simulink model "tasks_union_1"  (R2020b)
settings: Solver=FixedStepAuto  StartTime=0.0  StopTime=5  FixedStep=0.001  RelTol=1e-3
values from neighbouring files (symbols this model uses):
  a = evalin('base','a')    [Coriolis.m]    (also in init.m = 0.5)
  a0 = 0.99    [init.m]
  ac = mass_can*(l1*l2)    (= 0.5)    [init.m]
  berta = 0.98    [init.m]
  csi = 1    [init.m]
  e_max = 0.01    [init.m]
  F_int_max = [2;2]    [init.m]
  F_max = [2;2]    [init.m]
  F_weight = [0;-0.5*mass_can*g]    [init.m]
  g = evalin('base','g')    [Gravity.m]    (also in init.m = 9.81)
  I1 = evalin('base','I1')    [Mass.m]    (also in init.m = 1)
  I2 = evalin('base','I2')    [Mass.m]    (also in init.m = 1)
  Ic = mass_can*l2^2    (= 0.5)    [init.m]
  l1 = evalin('base','l1')    [Gravity.m]    (also in Jacobianoa_dot.m; Mass.m; cin_dir.m; init.m = 1)
  l2 = evalin('base','l2')    [Gravity.m]    (also in Jacobianoa_dot.m; Mass.m; cin_dir.m; init.m = 1)
  M = 0.1    [init.m]
  m1 = evalin('base','m1')    [Gravity.m]    (also in Mass.m; init.m = 1)
  m2 = evalin('base','m2')    [Gravity.m]    (also in Mass.m; init.m = 1)
  mass = 0.1    [init.m]
  mass_can = 0.5    [init.m]
libraries: simulink x1
settings Model: Creator=chiara-s  LastModifiedBy=chiara-s

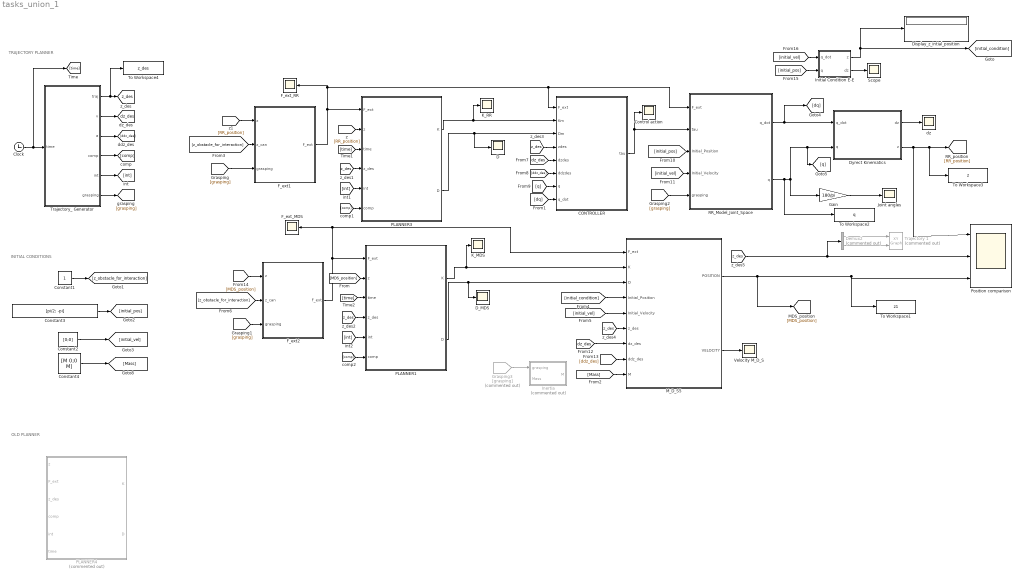
== system tasks_union_1 ==
  note: OLD PLANNER
  note: TRAJECTORY PLANNER
  note: INITIAL CONDITIONS
  CONTROLLER : MATLAB Function  TreatAsAtomicUnit=on
  Clock : Clock
  Constant1 : Constant
  Constant2 : Constant  Value=[0;0]
  Constant3 : Constant  Value=[pi/2; -pi]
  Constant4 : Constant  Value=[M 0;0 M]
  Control action : Scope
  D : Scope
  D_MDS : Scope
  Demux2 : Demux  Commented=on  Outputs=2
  Display_z_intial_position : Display
  Dyrect Kinematics : MATLAB Function  TreatAsAtomicUnit=on
  F_ext1 : MATLAB Function  TreatAsAtomicUnit=on
  F_ext2 : MATLAB Function  TreatAsAtomicUnit=on
  F_ext_MDS : Scope
  F_ext_RR : Scope
  Gain : Gain  Gain=180/pi
  Grasping3 : From  Commented=on  GotoTag=grasping
  "Inertia " : MATLAB Function  Commented=on  TreatAsAtomicUnit=on
  Initial Condition E-E : MATLAB Function  TreatAsAtomicUnit=on
  Joint angles : Scope
  K_MDS : Scope
  K_RR : Scope
  M_D_S5 : Subsystem
  PLANNER1 : Subsystem
  PLANNER3 : Subsystem
  PLANNER4 : Subsystem  Commented=on
  Position comparison : Scope  NumInputPorts=3
  RR_Model_Joint_Space : Subsystem
  Scope : Scope
  To Workspace1 : ToWorkspace  VariableName=z1  SaveFormat=Timeseries  SampleTime=-1
  To Workspace2 : ToWorkspace  VariableName=q  SaveFormat=Timeseries  SampleTime=-1
      settings: Save2DSignal=2-D array (concatenate along first dimension)
  To Workspace3 : ToWorkspace  VariableName=z  SaveFormat=Timeseries  SampleTime=-1
  To Workspace4 : ToWorkspace  VariableName=z_des  SaveFormat=Timeseries  SampleTime=-1
      settings: Save2DSignal=2-D array (concatenate along first dimension)
  Trajectory 1 : simulink/Sinks/XY Graph  Commented=on  xmin=-2  xmax=2  ymin=-2  ymax=2  st=-1
  Trajectory_ Generator : MATLAB Function  TreatAsAtomicUnit=on
  Velocity M_D_S : Scope
  dz : Scope
  tag scope: dz_des=global, z_des=global
  wires:
  Initial Condition E-E/1(z) -> Display_z_intial_position/1, [initial_condition]
  Initial Condition E-E/2(dz) -> Scope/1
  Gain/1 -> Joint angles/1
  Constant1/1 -> [z_obstacle_for_interaction]
  Constant2/1 -> [initial_vel]
  Constant3/1 -> [initial_pos]
  Constant4/1 -> [Mass]
  Clock/1 -> [time], Trajectory_ Generator/1(time)
  [z_obstacle_for_interaction] -> F_ext2/2(z_can)
  Trajectory_ Generator/1(traj) -> To Workspace4/1, [z_des]
  Trajectory_ Generator/2(v) -> [dz_des]
  Trajectory_ Generator/3(a) -> [ddz_des]
  Trajectory_ Generator/4(comp) -> [comp]
  Trajectory_ Generator/5(int) -> [int]
  Trajectory_ Generator/6(grasping) -> [grasping]
  [grasping] -> F_ext1/3(grasping)
  [grasping] -> F_ext2/3(grasping)
  [time] -> PLANNER3/3(time)
  [z_des] -> PLANNER1/4(z_des)
  [z_obstacle_for_interaction] -> F_ext1/2(z_can)
  [comp] -> PLANNER1/6(comp)
  [int] -> PLANNER3/5(int)
  [int] -> PLANNER1/5(int)
  [time] -> PLANNER1/3(time)
  RR_Model_Joint_Space/1(q_dot) -> [dq], Dyrect Kinematics/1(q_dot)
  RR_Model_Joint_Space/2(q) -> Gain/1, [q], Dyrect Kinematics/2(q), To Workspace2/1
  Dyrect Kinematics/1(dz) -> dz/1
  Dyrect Kinematics/2(z) -> Position comparison/1, To Workspace3/1, [RR_position]
  F_ext1/1(F_ext) -> PLANNER3/1(F_ext), RR_Model_Joint_Space/1(F_ext), CONTROLLER/1(F_ext), F_ext_RR/1
  [RR_position] -> F_ext1/1(z)
  CONTROLLER/1(tau) -> Control action/1, RR_Model_Joint_Space/2(tau)
  [z_des] -> CONTROLLER/4(zdes)
  [dz_des] -> CONTROLLER/5(dzdes)
  PLANNER3/1(K) -> K_RR/1, CONTROLLER/2(Km)
  PLANNER3/2(D) -> D/1, CONTROLLER/3(Dm)
  PLANNER1/1(K) -> K_MDS/1, M_D_S5/2(K)
  PLANNER1/2(D) -> D_MDS/1, M_D_S5/3(D)
  [ddz_des] -> CONTROLLER/6(ddzdes)
  [initial_pos] -> RR_Model_Joint_Space/3(Initial_Position)
  [initial_vel] -> RR_Model_Joint_Space/4(Initial_Velocity)
  [grasping] -> RR_Model_Joint_Space/5(grasping)
  [initial_condition] -> M_D_S5/4(Initial_Position)
  [initial_vel] -> M_D_S5/5(Initial_Velocity)
  Grasping3/1 -> "Inertia "/1(grasping)
  [z_des] -> M_D_S5/6(z_des)
  [dz_des] -> M_D_S5/7(dz_des)
  [ddz_des] -> M_D_S5/8(ddz_des)
  M_D_S5/2(VELOCITY) -> Velocity M_D_S/1
  M_D_S5/1(POSITION) -> [MDS_position], To Workspace1/1, Position comparison/3
  [z_des] -> Demux2/1, Position comparison/2
  Demux2/2 -> Trajectory 1/2
  Demux2/1 -> Trajectory 1/1
  [dq] -> CONTROLLER/8(q_dot)
  [q] -> CONTROLLER/7(q)
  [MDS_position] -> F_ext2/1(z)
  [initial_vel] -> Initial Condition E-E/1(q_dot)
  [initial_pos] -> Initial Condition E-E/2(q)
  F_ext2/1(F_ext) -> PLANNER1/1(F_ext), M_D_S5/1(F_ext), F_ext_MDS/1
  [Mass] -> M_D_S5/9(M)
  [RR_position] -> PLANNER3/2(z)
  [comp] -> PLANNER3/6(comp)
  [z_des] -> PLANNER3/4(z_des)
  [MDS_position] -> PLANNER1/2(z)

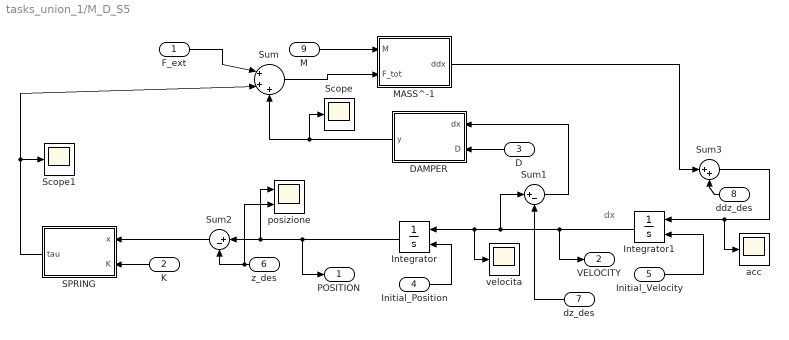
== system tasks_union_1/M_D_S5 ==
  note: dx
  F_ext : Inport
  K : Inport  Port=2
  D : Inport  Port=3
  Initial_Position : Inport  Port=4
  Initial_Velocity : Inport  Port=5
  z_des : Inport  Port=6
  dz_des : Inport  Port=7
  ddz_des : Inport  Port=8
  M : Inport  Port=9
  DAMPER : MATLAB Function  TreatAsAtomicUnit=on
  Integrator : Integrator  InitialConditionSource=external
  Integrator1 : Integrator  InitialConditionSource=external
  MASS^-1 : MATLAB Function  TreatAsAtomicUnit=on
  SPRING : MATLAB Function  TreatAsAtomicUnit=on
  Scope : Scope
  Scope1 : Scope
  Sum : Sum  Inputs=|+++
  Sum1 : Sum  Inputs=|+-
  Sum2 : Sum  Inputs=|+-
  Sum3 : Sum  Inputs=|++
  acc : Scope
  posizione : Scope  NumInputPorts=2
  velocita : Scope
  POSITION : Outport
  VELOCITY : Outport  Port=2
  wires:
  Integrator1/1 -> velocita/1, Integrator/1, Sum1/1, VELOCITY/1
  SPRING/1(tau) -> Sum/2, Scope1/1
  Integrator/1 -> posizione/1, Sum2/1, POSITION/1
  DAMPER/1(y) -> Scope/1, Sum/3
  Sum/1 -> MASS^-1/2(F_tot)
  M/1 -> MASS^-1/1(M)
  D/1 -> DAMPER/2(D)
  K/1 -> SPRING/2(K)
  Initial_Velocity/1 -> Integrator1/2
  Initial_Position/1 -> Integrator/2
  z_des/1 -> posizione/2, Sum2/2
  Sum2/1 -> SPRING/1(x)
  MASS^-1/1(ddx) -> Sum3/1
  Sum1/1 -> DAMPER/1(dx)
  Sum3/1 -> acc/1, Integrator1/1
  dz_des/1 -> Sum1/2
  ddz_des/1 -> Sum3/2
  F_ext/1 -> Sum/1

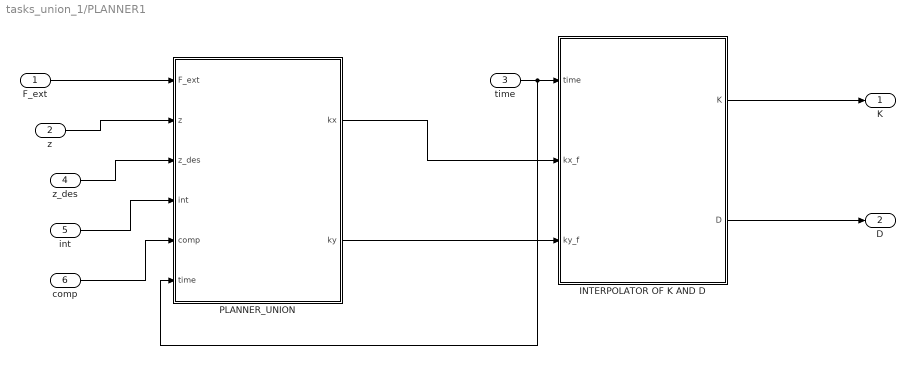
== system tasks_union_1/PLANNER1 ==
  F_ext : Inport
  z : Inport  Port=2
  time : Inport  Port=3
  z_des : Inport  Port=4
  int : Inport  Port=5
  comp : Inport  Port=6
  "INTERPOLATOR OF K AND D " : MATLAB Function  TreatAsAtomicUnit=on
  PLANNER_UNION : MATLAB Function  TreatAsAtomicUnit=on
  K : Outport
  D : Outport  Port=2
  wires:
  time/1 -> "INTERPOLATOR OF K AND D "/1(time), PLANNER_UNION/6(time)
  "INTERPOLATOR OF K AND D "/2(D) -> D/1
  "INTERPOLATOR OF K AND D "/1(K) -> K/1
  PLANNER_UNION/2(ky) -> "INTERPOLATOR OF K AND D "/3(ky_f)
  PLANNER_UNION/1(kx) -> "INTERPOLATOR OF K AND D "/2(kx_f)
  int/1 -> PLANNER_UNION/4(int)
  comp/1 -> PLANNER_UNION/5(comp)
  F_ext/1 -> PLANNER_UNION/1(F_ext)
  z/1 -> PLANNER_UNION/2(z)
  z_des/1 -> PLANNER_UNION/3(z_des)

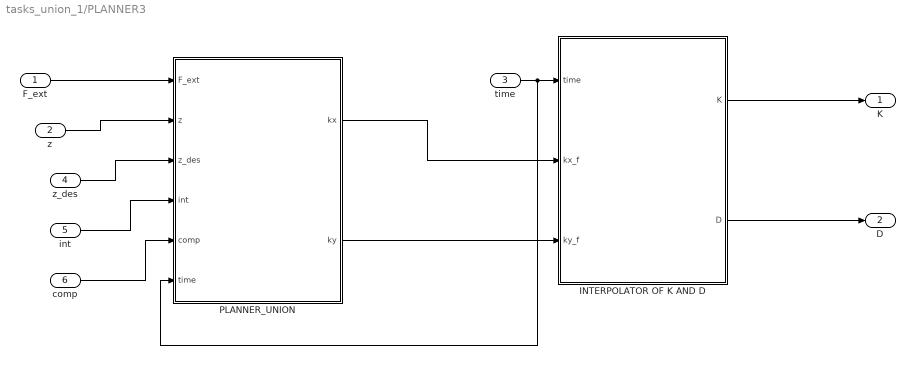
== system tasks_union_1/PLANNER3 ==
  F_ext : Inport
  z : Inport  Port=2
  time : Inport  Port=3
  z_des : Inport  Port=4
  int : Inport  Port=5
  comp : Inport  Port=6
  "INTERPOLATOR OF K AND D " : MATLAB Function  TreatAsAtomicUnit=on
  PLANNER_UNION : MATLAB Function  TreatAsAtomicUnit=on
  K : Outport
  D : Outport  Port=2
  wires:
  time/1 -> "INTERPOLATOR OF K AND D "/1(time), PLANNER_UNION/6(time)
  "INTERPOLATOR OF K AND D "/2(D) -> D/1
  "INTERPOLATOR OF K AND D "/1(K) -> K/1
  PLANNER_UNION/2(ky) -> "INTERPOLATOR OF K AND D "/3(ky_f)
  PLANNER_UNION/1(kx) -> "INTERPOLATOR OF K AND D "/2(kx_f)
  int/1 -> PLANNER_UNION/4(int)
  comp/1 -> PLANNER_UNION/5(comp)
  F_ext/1 -> PLANNER_UNION/1(F_ext)
  z/1 -> PLANNER_UNION/2(z)
  z_des/1 -> PLANNER_UNION/3(z_des)

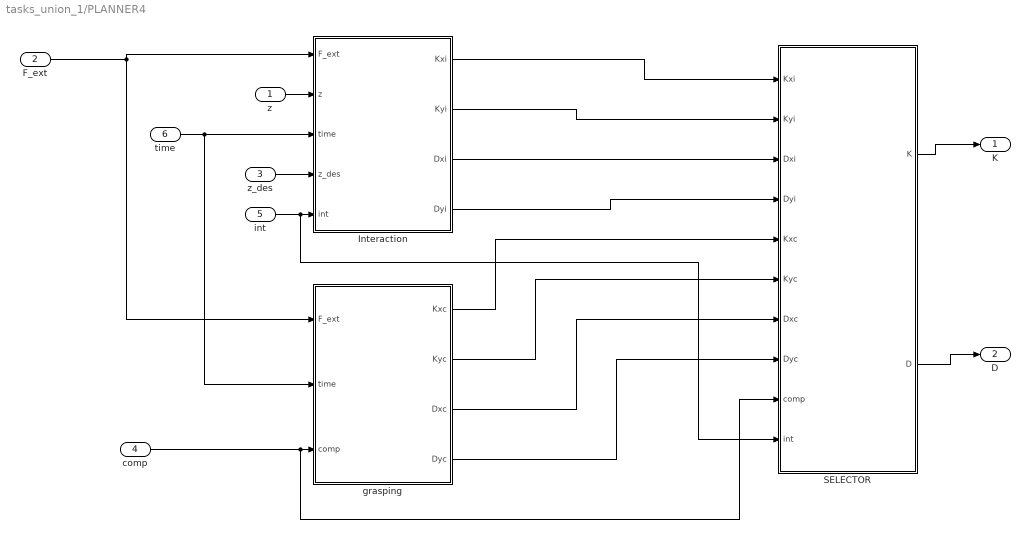
== system tasks_union_1/PLANNER4 ==
  z : Inport
  F_ext : Inport  Port=2
  z_des : Inport  Port=3
  comp : Inport  Port=4
  int : Inport  Port=5
  time : Inport  Port=6
  Interaction : MATLAB Function  TreatAsAtomicUnit=on
  SELECTOR : MATLAB Function  TreatAsAtomicUnit=on
  grasping : MATLAB Function  TreatAsAtomicUnit=on
  K : Outport
  D : Outport  Port=2
  wires:
  time/1 -> grasping/2(time), Interaction/3(time)
  z_des/1 -> Interaction/4(z_des)
  F_ext/1 -> grasping/1(F_ext), Interaction/1(F_ext)
  z/1 -> Interaction/2(z)
  SELECTOR/1(K) -> K/1
  SELECTOR/2(D) -> D/1
  Interaction/1(Kxi) -> SELECTOR/1(Kxi)
  Interaction/2(Kyi) -> SELECTOR/2(Kyi)
  Interaction/3(Dxi) -> SELECTOR/3(Dxi)
  Interaction/4(Dyi) -> SELECTOR/4(Dyi)
  grasping/1(Kxc) -> SELECTOR/5(Kxc)
  grasping/2(Kyc) -> SELECTOR/6(Kyc)
  grasping/3(Dxc) -> SELECTOR/7(Dxc)
  grasping/4(Dyc) -> SELECTOR/8(Dyc)
  comp/1 -> SELECTOR/9(comp), grasping/3(comp)
  int/1 -> SELECTOR/10(int), Interaction/5(int)

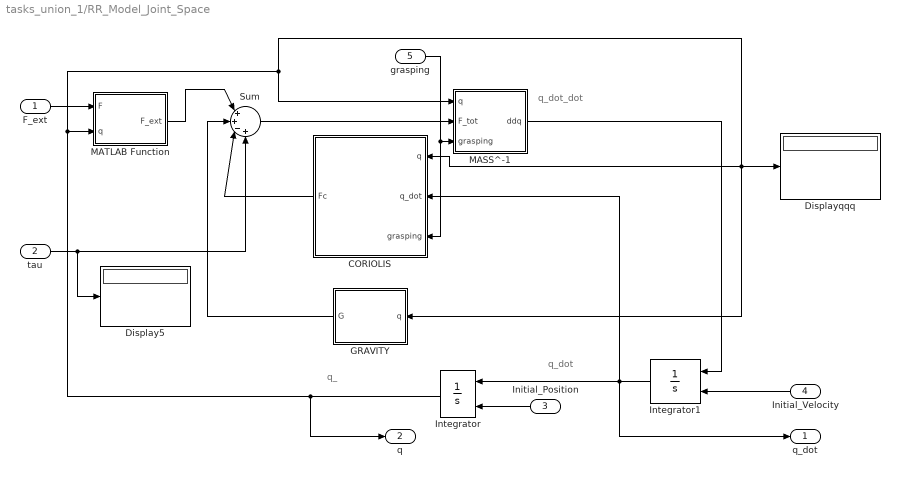
== system tasks_union_1/RR_Model_Joint_Space ==
  note: q_dot
  note: q_dot_dot
  note: q_
  F_ext : Inport
  tau : Inport  Port=2
  Initial_Position : Inport  Port=3
  Initial_Velocity : Inport  Port=4
  grasping : Inport  Port=5
  CORIOLIS : MATLAB Function  TreatAsAtomicUnit=on
  Display5 : Display
  Displayqqq : Display
  GRAVITY : MATLAB Function  TreatAsAtomicUnit=on
  Integrator : Integrator  InitialConditionSource=external
  Integrator1 : Integrator  InitialConditionSource=external  InitialCondition=[0;0]
  MASS^-1 : MATLAB Function  TreatAsAtomicUnit=on
  MATLAB Function : MATLAB Function  TreatAsAtomicUnit=on
  Sum : Sum  Inputs=|++-+
  q_dot : Outport
  q : Outport  Port=2
  wires:
  GRAVITY/1(G) -> Sum/2
  MATLAB Function/1(F_ext) -> Sum/1
  Initial_Position/1 -> Integrator/2
  F_ext/1 -> MATLAB Function/1(F)
  Integrator/1 -> MASS^-1/1(q), GRAVITY/1(q), Displayqqq/1, CORIOLIS/1(q), MATLAB Function/2(q), q/1
  Integrator1/1 -> q_dot/1, CORIOLIS/2(q_dot), Integrator/1
  Initial_Velocity/1 -> Integrator1/2
  MASS^-1/1(ddq) -> Integrator1/1
  Sum/1 -> MASS^-1/2(F_tot)
  CORIOLIS/1(Fc) -> Sum/3
  tau/1 -> Display5/1, Sum/4
  grasping/1 -> CORIOLIS/3(grasping), MASS^-1/3(grasping)

== matlab function tasks_union_1/Dyrect Kinematics ==
  data: q_dot input double size=2; dz output double size=2; q input double size=2; z output double size=2; l1 parameter; l2 parameter
function [dz,z] = fcn(q_dot,q,l1, l2)

z = zeros(2,1);
z(1) = l1*cos(q(1)) + l2*cos(q(1)+q(2));
z(2) = l1*sin(q(1)) + l2*sin(q(1)+q(2));

Ja = zeros(2,2);
Ja = [-l1*sin(q(1)) - l2*sin(q(1)+q(2)), -l2*sin(q(1)+q(2)); ...
    l1*cos(q(1)) + l2*cos(q(1)+q(2)), l2*cos(q(1)+q(2))];

dz = zeros(2,1);
dz = Ja*q_dot;

end

== matlab function tasks_union_1/PLANNER1/PLANNER_UNION ==
  settings: updateMethod=DISCRETE
  data: kx output; F_ext input; z input; z_des input; int input; comp input; ky output; e_max parameter; F_max parameter; F_int_max parameter; time input
function [kx, ky] = fcn(F_ext, z, z_des, int, comp, e_max, F_max, F_int_max, time)
%% Description MDS_interaction


%% Outputs
% K            stiffness 
% D            damping 

%% Inputs
% time          current simulation time
% F_ext         measured external force
% mass          mass scalar value 
% F_int_max     desired interaction force
% z_des         desired trajectory
% z             current position
% F_max         estimated force disturbances
% e_max         maximum steady-state error

persistent kxi kyi kxc kyc F_comp
persistent int_prec comp_prec z_int z_int_dir 

% persistent initialization
if isempty(kxi)
   kxi = F_max(1)/e_max; 
end
if isempty(F_comp)
   F_comp = [0;0];
end

if isempty(kyi)
   kyi = F_max(2)/e_max;
end
if isempty(kxc)
      kxc = F_max(1)/e_max;
end
if isempty(kyc)
      kyc = F_max(2)/e_max;
end
if isempty(z_int) 
    z_int = [1000; 1000];
end
if isempty(z_int_dir) 
    z_int_dir = [0;0];
end
if isempty(int_prec)
    int_prec = [0;0];
end
if isempty(comp_prec)
    comp_prec = [0;0];
end

% interaction X axes
if int(1) == 1
    if abs(F_ext(1)-F_comp(1)) > F_max(1)         % F_max soglia dei disturbi
        if z_int(1) == 1000
            z_int(1) = z(1);
            z_int_dir(1) = -sign(F_ext(1)-F_comp(1));     % direzione non permessa
        end
    end
    if abs(F_ext(1)-F_comp(1)) > F_int_max(1) 
            % if interaction force is higher than threshold
            if kxi*abs(z(1)-z_des(1)) > F_int_max(1)
                % set k 
                ktemp_x = F_int_max(1)/abs(z(1)-z_des(1));
                if ktemp_x < kxi
                    kxi = ktemp_x;
                end
            end
    end
end

% interaction Y axes
if int(2) == 1
    if abs(F_ext(2)-F_comp(2)) > F_max(2)         % F_max soglia dei disturbi
        if z_int(2) == 1000
            z_int(2) = z(2);
            z_int_dir(2) = -sign(F_ext(2)-F_comp(2));     % direzione non permessa
        end
    end
    % Similarly for the other direction
    if abs(F_ext(2)-F_comp(2)) > F_int_max(2) 
            if kyi*abs(z(2)-z_des(2)) > F_int_max(2)
                ktemp_y = F_int_max(2)/abs(z(2)-z_des(2));
                if ktemp_y < kyi
                    kyi = ktemp_y;
                end
            end
    end
end

% compensation X axes
if comp(1) == 1
    if z_int(1) == 1000
       if abs(F_ext(1))/kxc > e_max
            kxc = abs(F_ext(1))/e_max;
            F_comp(1) = F_ext(1);
       end
    else 
        if z_int_dir(1) == 1
            if z(1) < z_int(1)
                if abs(F_ext(1))/kxc > e_max 
                    kxc = abs(F_ext(1))/e_max;
                    F_comp(1) = F_ext(1);
                end
            end
        else
            if z(1) > z_int(1)
                if abs(F_ext(1))/kxc > e_max
                    kxc = abs(F_ext(1))/e_max;
                    F_comp(1) = F_ext(1);
                end
            end
        end
                
   end
end

% compensation Y axes
if comp(2) == 1
    if z_int(2) == 1000 
       if abs(F_ext(2))/kyc > e_max
            kyc = abs(F_ext(2))/e_max;
            F_comp(2) = F_ext(2);
       end
    else 
        if z_int_dir(2) == 1
            if z(2) < z_int(2)
                if abs(F_ext(2))/kyc > e_max
                    kyc = abs(F_ext(2))/e_max;
                    F_comp(2) = F_ext(2);
                end
            end
        else
            if z(2) > z_int(2)
                if abs(F_ext(2))/kyc > e_max
                    kyc = abs(F_ext(2))/e_max;
                    F_comp(2) = F_ext(2);
                end
            end
        end
                
   end
end

% reset to default
if comp(1)==0 && comp_prec(1)==1
%     z_int_dir(1) = 0;
%     z_int(1) = 1000;
    kxc = F_max(1)/e_max;
    F_comp(1) = 0;
end
if comp(2)==0 && comp_prec(2)==1
%     z_int_dir(2) = 0;
%     z_int(2) = 1000;
    kyc = F_max(2)/e_max;
    F_comp(2) = 0;
end
if int(1)==0 && int_prec(1)==1
    kxi = F_max(1)/e_max;
end
if int(2)==0 && int_prec(2)==1
    kyi = F_max(2)/e_max;
end
% quando c'è una interazione e prima non c'era risetto tutto (RACCAPEZZO)
if int(1)==1 && int_prec(1)==0
    if comp_prec(1) == 1
        kxi = kxc;
    end
    z_int(1)=1000;
    z_int_dir(1)=0;
end
if int(2)==1 && int_prec(2)==0
    if comp_prec(2) == 1
        kyi = kyc;
    end
    z_int(2)=1000;
    z_int_dir(2)=0;
end
if comp(1) == 1 && comp_prec(1)==0
    if int_prec(1) == 1
        kxc = kxi;
    end
end
if comp(2) == 1 && comp_prec(2)==0
    if int_prec(2)==1
        kyc =kyi;
    end
end
% update last booleans
int_prec = int;
comp_prec = comp;


% Final Values of D-K
kx = abs(F_max(1))/e_max;
ky = abs(F_max(2))/e_max;

if comp(1) == 1
    kx = kxc;
end
if comp(2) == 1
    ky = kyc;
end
if int(1) == 1
    kx = kxi;
    if comp(1) == 1
        if z_int(1) == 1000
            kx = kxc;
        else
            if z_int_dir(1) == 1
                if z_des(1) < z_int(1)
                    kx = kxc;
                end
            else
                if z_des(1) > z_int(1)
                    kx = kxc;
                end
            end
        end
    else
        if z_int(1) == 1000
            kx = F_max(1)/e_max;
        else
            if z_int_dir(1) == 1
                if z_des(1) < z_int(1)
                    kx = F_max(1)/e_max;
                end
            else
                if z_des(1) > z_int(1)
                    kx = F_max(1)/e_max;
                end
            end
        end
    end
end
if int(2) == 1
    ky = kyi;
     if comp(2) == 1
        if z_int(2) == 1000
            kx = kxc;
        else
            if z_int_dir(2) == 1
                if z_des(2) < z_int(2) 
                    ky = kyc;
                end
            else
                if z_des(2) > z_int(2)
                    ky = kyc;
                end
            end
        end
     else
         if z_int(2) == 1000
            kx = F_max(2)/e_max;
        else
            if z_int_dir(2) == 1
                if z_des(2) < z_int(2) 
                    ky = F_max(2)/e_max;
                end
            else
                if z_des(2) > z_int(2)
                    ky = F_max(2)/e_max;
                end
            end
        end
     end
end

end

== matlab function tasks_union_1/Trajectory_ Generator ==
  data: time input; traj output; v output; a output; comp output; int output; grasping output
function [traj,v, a, comp, int, grasping] = fcn(time)

comp = [0;0];
int = [0;0];
t_prec = 0;
grasping = 0;

if time < 0.1
    a = [5;0];
    traj = 0.5*a*(time)^2;   % initial vel = 0;
    v = a*time;
    int(1) = 1;
elseif time < 2.3
    v = [0.5;0];
    x0 = [0.025;0];
    traj = x0 + v*(time-0.1); 
    a = [0;0];
    int(1) = 1;
elseif time < 2.4
    a = [-5;0];
    x0 = [1.125;0];
    v0 = [0.5;0];
    v = v0 + a*(time -2.3);
    traj = x0 + 0.5*a*(time -2.3)^2 + v0*(time-2.3);
    int(1) = 1;
elseif time < 3
    int(1) = 1;
    traj = [1.15;0];  
    a = [0;0];
    v = [0;0];
elseif time < 3.1
    a = [0; 5];
    v = a*(time-3);
    x0 = [1.15;0];
    traj = 0.5*a*(time -3)^2 + x0;
    comp(2) = 1;
    int(1) = 1;
    grasping = 1;
elseif time < 4.1
    comp(2) = 1;
    v = [0; 0.5];
    x0 = [1.15;0.025];
    traj = x0 + v*(time-3.1);
    a = [0;0];
    grasping = 1;
    int(1) = 1;
elseif time < 4.2
    comp(2) = 1;
    a = [0; -5];
    x0 = [1.15; 0.525];
    v0 = [0; 0.5];
    v = v0 +a*(time-4.1);
    traj = x0 + 0.5*a*(time-4.1)^2 + v0*(time-4.1);
    grasping = 1;
else
    traj = [1.15; 0.55];
    comp(2) = 1;
    a = [0;0];
    v = [0;0];
    grasping = 1;
end

end

== matlab function tasks_union_1/F_ext1 ==
  data: z input; F_ext output; z_can input; grasping input; mass_can parameter; g parameter
function F_ext = fcn(z, z_can, grasping, mass_can, g)
% hypothesis: table reaction force with elastic behaviour
F_ext = zeros(2,1);
k_can = 500;         
k_table = 10000;
% if contact is happened with can
if grasping == 0
    if z(1) > z_can
        F_ext(1) = k_can*(z_can - z(1));    % force to the left
    end
else 
    F_ext(1) = 0;
    F_ext(2) = -mass_can*g;
    if z(2) < 0
         F_ext(2) = - k_table*z(2);       % in grasping on the table
    else 
        if (abs(k_table*z(2)) < abs(mass_can*g))
            F_ext(2) = - k_table*z(2);
        else 
            F_ext(2) = - mass_can*g;        % STACCATO
        end    
    end
end
end

== matlab function tasks_union_1/Inertia  ==
  data: M output; grasping input; mass_can parameter; Mass input
function M = fcn(grasping, mass_can, Mass)

if grasping == 1
    M = diag([Mass(1,1)+mass_can Mass(2,2)+mass_can]);
else
    M = Mass;
end

end

== matlab function tasks_union_1/CONTROLLER ==
  data: F_ext input; Km input; Dm input; zdes input size=2; tau output double size=2; dzdes input size=2; ddzdes input size=2; q input size=2; q_dot input size=2; M parameter
function tau = fcn(F_ext,Km, Dm,zdes, dzdes, ddzdes, q, q_dot, M)
%% PROBLEMA MATRICE DELLE MASSE NON DIAGONALE
coder.extrinsic('Jacobianoa','Jacobianoa_dot','Mass','Coriolis','Gravity','cin_dir')
dz = zeros(2,1);
z = zeros(2,1);
B = zeros(2,2);
S = zeros(2,2);
G = zeros(2,1);
Ja = zeros(2,2);
Ja_dot = zeros(2,2);
Bm = [M 0; 0 M];
Ja = Jacobianoa(q);
Ja_dot = Jacobianoa_dot(q,q_dot);

dz = Ja*q_dot;
z = cin_dir(q);

t = 0.1;
if (deg2rad(-0.1) < q(2)) && (q(2) < deg2rad(0.1)) || (deg2rad(179.9) < q(2)) && (q(2) < deg2rad(180.1)) || (deg2rad(-180.1) < q(2)) && (q(2) < deg2rad(-179.9))
    Ja_inv = (Ja')*inv(Ja*(Ja') + t^2*eye(2,2)); % Damp least square Jacobian method
else 
    Ja_inv = inv(Ja);
end

% Ja_inv = inv(Ja);

B = Mass(q);
Bx = (Ja_inv')* B * Ja_inv;
S = Coriolis(q,q_dot);
G = Gravity(q);
I = eye(2,2);
% tau = B * Ja_inv*(ddzdes - Ja_dot*q_dot) + ...
%     S*q_dot + (Ja')*(Dm*(dzdes - dz) + Km*(zdes- z)) + G;

tau = B*Ja_inv*(ddzdes - Ja_dot*q_dot + ...
    inv(Bm)*(Dm*(dzdes - dz) + Km*(zdes- z))) + S*q_dot - G + ...
    (Ja')*(Bx*inv(Bm) - I)*F_ext;

end

== matlab function tasks_union_1/Initial Condition E-E ==
  data: q_dot input double size=2; q input double size=2; z output double size=2; dz output double size=2; l1 parameter; l2 parameter
function [z,dz] = fcn(q_dot,q,l1, l2)

z = zeros(2,1);
z(1) = l1*cos(q(1)) + l2*cos(q(1)+q(2));
z(2) = l1*sin(q(1)) + l2*sin(q(1)+q(2));

Ja = zeros(2,2);
Ja = [-l1*sin(q(1)) - l2*sin(q(1)+q(2)), -l2*sin(q(1)+q(2)); ...
    l1*cos(q(1)) + l2*cos(q(1)+q(2)), l2*cos(q(1)+q(2))];

dz = zeros(2,1);
dz = Ja*q_dot;

end

== matlab function tasks_union_1/PLANNER3/INTERPOLATOR OF K AND D  ==
  settings: updateMethod=DISCRETE
  data: time input; K output; kx_f input; ky_f input; D output; e_max parameter; F_max parameter; M parameter; berta parameter; a0 parameter; mass parameter; csi parameter
function [K,D] = fcn(time, kx_f, ky_f, e_max, F_max,M, berta, a0, mass, csi)

persistent kx ky time_prec

if isempty(time_prec)
    time_prec = 0;
end

if isempty(kx)
   kx = F_max(1)/e_max; 
end
if isempty(ky)
   ky = F_max(2)/e_max;
end

% everytime k is increasing in accordance with stability condition
if kx_f <= kx
    kx = kx_f;
else 
    kx_i = kx;
    k_dotx = berta*(4*a0*sqrt(kx_i/mass)*(kx_i)^(3/2))/(sqrt(kx_i) + 2*a0*csi*sqrt(kx_i));
    k_tempx = kx_i + k_dotx*(time -time_prec);
    if k_tempx > kx_f
        kx = kx_f;
    else
        kx = k_tempx;
    end
end

if ky_f <= ky
    ky = ky_f;
else 
    ky_i = ky;
    k_doty = berta*(4*a0*sqrt(ky_i/mass)*(ky_i)^(3/2))/(sqrt(ky_i) + 2*a0*csi*sqrt(ky_i));
    k_tempy = ky_i + k_doty*(time -time_prec);
    if k_tempy > ky_f
        ky = ky_f;
    else
        ky = k_tempy;
    end
end
time_prec = time;

dx = sqrt(4*kx*M);
dy = sqrt(4*ky*M);

D = diag([dx,dy]);
K = diag([kx,ky]);

end

== matlab function tasks_union_1/PLANNER3/PLANNER_UNION ==
  settings: updateMethod=DISCRETE
  data: kx output; F_ext input; z input; z_des input; int input; comp input; ky output; e_max parameter; F_max parameter; F_int_max parameter; time input
function [kx, ky] = fcn(F_ext, z, z_des, int, comp, e_max, F_max, F_int_max, time)
%% Description MDS_interaction


%% Outputs
% K            stiffness 
% D            damping 

%% Inputs
% time          current simulation time
% F_ext         measured external force
% mass          mass scalar value 
% F_int_max     desired interaction force
% z_des         desired trajectory
% z             current position
% F_max         estimated force disturbances
% e_max         maximum steady-state error

persistent kxi kyi kxc kyc F_comp
persistent int_prec comp_prec z_int z_int_dir 

% persistent initialization
if isempty(kxi)
   kxi = F_max(1)/e_max; 
end
if isempty(F_comp)
   F_comp = [0;0];
end

if isempty(kyi)
   kyi = F_max(2)/e_max;
end
if isempty(kxc)
      kxc = F_max(1)/e_max;
end
if isempty(kyc)
      kyc = F_max(2)/e_max;
end
if isempty(z_int) 
    z_int = [1000; 1000];
end
if isempty(z_int_dir) 
    z_int_dir = [0;0];
end
if isempty(int_prec)
    int_prec = [0;0];
end
if isempty(comp_prec)
    comp_prec = [0;0];
end

% interaction X axes
if int(1) == 1
    if abs(F_ext(1)-F_comp(1)) > F_max(1)         % F_max soglia dei disturbi
        if z_int(1) == 1000
            z_int(1) = z(1);
            z_int_dir(1) = -sign(F_ext(1)-F_comp(1));     % direzione non permessa
        end
    end
    if abs(F_ext(1)-F_comp(1)) > F_int_max(1) 
            % if interaction force is higher than threshold
            if kxi*abs(z(1)-z_des(1)) > F_int_max(1)
                % set k 
                ktemp_x = F_int_max(1)/abs(z(1)-z_des(1));
                if ktemp_x < kxi
                    kxi = ktemp_x;
                end
            end
    end
end

% interaction Y axes
if int(2) == 1
    if abs(F_ext(2)-F_comp(2)) > F_max(2)         % F_max soglia dei disturbi
        if z_int(2) == 1000
            z_int(2) = z(2);
            z_int_dir(2) = -sign(F_ext(2)-F_comp(2));     % direzione non permessa
        end
    end
    % Similarly for the other direction
    if abs(F_ext(2)-F_comp(2)) > F_int_max(2) 
            if kyi*abs(z(2)-z_des(2)) > F_int_max(2)
                ktemp_y = F_int_max(2)/abs(z(2)-z_des(2));
                if ktemp_y < kyi
                    kyi = ktemp_y;
                end
            end
    end
end

% compensation X axes
if comp(1) == 1
    if z_int(1) == 1000
       if abs(F_ext(1))/kxc > e_max
            kxc = abs(F_ext(1))/e_max;
            F_comp(1) = F_ext(1);
       end
    else 
        if z_int_dir(1) == 1
            if z(1) < z_int(1)
                if abs(F_ext(1))/kxc > e_max 
                    kxc = abs(F_ext(1))/e_max;
                    F_comp(1) = F_ext(1);
                end
            end
        else
            if z(1) > z_int(1)
                if abs(F_ext(1))/kxc > e_max
                    kxc = abs(F_ext(1))/e_max;
                    F_comp(1) = F_ext(1);
                end
            end
        end
                
   end
end

% compensation Y axes
if comp(2) == 1
    if z_int(2) == 1000 
       if abs(F_ext(2))/kyc > e_max
            kyc = abs(F_ext(2))/e_max;
            F_comp(2) = F_ext(2);
       end
    else 
        if z_int_dir(2) == 1
            if z(2) < z_int(2)
                if abs(F_ext(2))/kyc > e_max
                    kyc = abs(F_ext(2))/e_max;
                    F_comp(2) = F_ext(2);
                end
            end
        else
            if z(2) > z_int(2)
                if abs(F_ext(2))/kyc > e_max
                    kyc = abs(F_ext(2))/e_max;
                    F_comp(2) = F_ext(2);
                end
            end
        end
                
   end
end

% reset to default
if comp(1)==0 && comp_prec(1)==1
%     z_int_dir(1) = 0;
%     z_int(1) = 1000;
    kxc = F_max(1)/e_max;
    F_comp(1) = 0;
end
if comp(2)==0 && comp_prec(2)==1
%     z_int_dir(2) = 0;
%     z_int(2) = 1000;
    kyc = F_max(2)/e_max;
    F_comp(2) = 0;
end
if int(1)==0 && int_prec(1)==1
    kxi = F_max(1)/e_max;
end
if int(2)==0 && int_prec(2)==1
    kyi = F_max(2)/e_max;
end
% quando c'è una interazione e prima non c'era risetto tutto (RACCAPEZZO)
if int(1)==1 && int_prec(1)==0
    if comp_prec(1) == 1
        kxi = kxc;
    end
    z_int(1)=1000;
    z_int_dir(1)=0;
end
if int(2)==1 && int_prec(2)==0
    if comp_prec(2) == 1
        kyi = kyc;
    end
    z_int(2)=1000;
    z_int_dir(2)=0;
end
if comp(1) == 1 && comp_prec(1)==0
    if int_prec(1) == 1
        kxc = kxi;
    end
end
if comp(2) == 1 && comp_prec(2)==0
    if int_prec(2)==1
        kyc =kyi;
    end
end
% update last booleans
int_prec = int;
comp_prec = comp;


% Final Values of D-K
kx = abs(F_max(1))/e_max;
ky = abs(F_max(2))/e_max;

if comp(1) == 1
    kx = kxc;
end
if comp(2) == 1
    ky = kyc;
end
if int(1) == 1
    kx = kxi;
    if comp(1) == 1
        if z_int(1) == 1000
            kx = kxc;
        else
            if z_int_dir(1) == 1
                if z_des(1) < z_int(1)
                    kx = kxc;
                end
            else
                if z_des(1) > z_int(1)
                    kx = kxc;
                end
            end
        end
    else
        if z_int(1) == 1000
            kx = F_max(1)/e_max;
        else
            if z_int_dir(1) == 1
                if z_des(1) < z_int(1)
                    kx = F_max(1)/e_max;
                end
            else
                if z_des(1) > z_int(1)
                    kx = F_max(1)/e_max;
                end
            end
        end
    end
end
if int(2) == 1
    ky = kyi;
     if comp(2) == 1
        if z_int(2) == 1000
            kx = kxc;
        else
            if z_int_dir(2) == 1
                if z_des(2) < z_int(2) 
                    ky = kyc;
                end
            else
                if z_des(2) > z_int(2)
                    ky = kyc;
                end
            end
        end
     else
         if z_int(2) == 1000
            kx = F_max(2)/e_max;
        else
            if z_int_dir(2) == 1
                if z_des(2) < z_int(2) 
                    ky = F_max(2)/e_max;
                end
            else
                if z_des(2) > z_int(2)
                    ky = F_max(2)/e_max;
                end
            end
        end
     end
end

end

== matlab function tasks_union_1/RR_Model_Joint_Space/CORIOLIS ==
  data: q input size=2; Fc output double size=2; q_dot input size=2; a parameter; ac parameter; grasping input
function Fc = fcn(q,q_dot,a, ac, grasping)

C = zeros(2,2);
C = [-a*sin(q(2))*q_dot(2), -a*sin(q(2))*q_dot(1)-a*sin(q(2)*q_dot(2)); ...
    a*sin(q(2))*q_dot(1), 0];
% if grasping == 1
%     Cc = [-ac*sin(q(2))*q_dot(2), -ac*sin(q(2))*q_dot(1)-ac*sin(q(2)*q_dot(2)); ...
%           ac*sin(q(2))*q_dot(1), 0];
%       C =  C + Cc;
% end

Fc = C*q_dot;

end

== matlab function tasks_union_1/PLANNER4/Interaction ==
  settings: updateMethod=DISCRETE
  data: F_max parameter; Kxi output; Kyi output; e_max parameter; F_ext input; z input; time input; z_des input; F_int_max parameter; mass parameter; Dxi output; Dyi output; int input
function [Kxi,Kyi,Dxi,Dyi] = fcn(F_max, e_max,F_ext, z, time, z_des, F_int_max, mass, int)

%% Description MDS_interaction
% decrease k after contact is sensed to limit the interaction force

%% Outputs
% K            stiffness 
% D            damping 

%% Inputs
% time          current simulation time
% F_ext         measured external force
% mass          mass scalar value 
% F_int_max     desired interaction force
% z_des         desired trajectory
% z             current position
% F_max         estimated force disturbances
% e_max         maximum steady-state error

persistent F_prec kx ky dx dy t_changex t_changey t_interaction

% time of a first interaction
if isempty(t_interaction)
    t_interaction = 1000;
end

% time of last stiffness update
if isempty(t_changex)
    t_changex = 1000;
end
if isempty(t_changey)
    t_changey = 1000;
end

% previous measured force
if isempty(F_prec)
    F_prec = [0;0];
end

% initialization of k and d 
if isempty(kx)
   kx = F_max(1)/e_max; 
end
if isempty(ky)
   ky = F_max(2)/e_max;
end
if isempty(dx)
    dx = sqrt(4*kx*mass);
end
if isempty(dy)
    dy = sqrt(4*ky*mass);
end

if int(1) == 1
    if abs(F_ext(1)) > F_int_max(1) 
        % if force is increasing
%         if abs(F_prec(1)) < abs(F_ext(1))
            % if interaction force is higher than threshold
            if kx*abs(z(1)-z_des(1)) > F_int_max(1)
                % set k 
                ktemp_x = F_int_max(1)/abs(z(1)-z_des(1));
                if ktemp_x < kx
                    kx = ktemp_x;
                    dx = sqrt(4*kx*mass);
                end

%             end
        end
    end
end
if int(2) == 1
    
    % Similarly for the other direction
    if abs(F_ext(2)) > F_int_max(2) 
%         if abs(F_prec(2)) < abs(F_ext(2))
            if ky*abs(z(2)-z_des(2)) > F_int_max(2)
                ktemp_y = F_int_max(2)/abs(z(2)-z_des(2));
                if ktemp_y < ky
                    ky = ktemp_y;
                    dy = sqrt(4*ky*mass);
                end
%             end
        end
    end
end

% F_prec = F_ext;     % update for last force

% set final values 
Kxi = kx; 
Kyi = ky;
Dxi = dx;
Dyi = dy;
end

== matlab function tasks_union_1/M_D_S5/DAMPER ==
  data: dx input; y output; D input
function y = fcn(dx, D)
y = - D*dx;
end

== matlab function tasks_union_1/M_D_S5/MASS^-1 ==
  data: M input; ddx output; F_tot input
function ddx = fcn(M,F_tot)
ddx = (M^-1)*F_tot;
end

== matlab function tasks_union_1/M_D_S5/SPRING ==
  data: x input; tau output; K input
function tau = fcn(x, K)
tau= -K*x;
end

== matlab function tasks_union_1/PLANNER4/SELECTOR ==
  data: Kxi input; K output; Kyi input; Dxi input; Dyi input; Kxc input; Kyc input; Dxc input; Dyc input; comp input; int input; D output; M parameter; F_max parameter; e_max parameter
function [K,D] = fcn(Kxi,Kyi,Dxi,Dyi,Kxc,Kyc,Dxc,Dyc,comp,int, M, F_max, e_max)

K1 = F_max(1)/e_max; 
K2 = F_max(2)/e_max; 
D1 = sqrt(4*(F_max(1)/e_max)*M); 
D2 = sqrt(4*(F_max(2)/e_max)*M);

if comp(1) == 1
    K1 = Kxc;
    D1 = Dxc;
end

if comp(2) == 1
    K2 = Kyc;
    D2 = Dyc;
end

if int(1) == 1
    K1 = Kxi;
    D1 = Dxi;
end

if int(2) == 1
    K2 = Kyi;
    D2 = Dyi;
end

K = diag([K1 K2]);
D = diag([D1 D2]);

end

== matlab function tasks_union_1/PLANNER4/grasping ==
  settings: updateMethod=DISCRETE
  data: Kxc output; Kyc output; e_max parameter; F_ext input; mass parameter; F_weight parameter; time input; a0 parameter; csi parameter; berta parameter; Dxc output; Dyc output; F_max parameter; comp input
function [Kxc,Kyc,Dxc,Dyc] = fcn(e_max, F_ext, mass, F_weight, time, a0, csi, berta, F_max, comp)

%% need to add reset of k after comp is zero. 

% with an estimated weight, k and d increase 
%% Outputs
% Km            stiffness matrix
% Dm            damping matrix 
%% Inputs
% time          current simulation time
% F_ext         measured external force

% variables initialization 
persistent kx_i ky_i dx dy timeG kx ky F_grasp kx_f ky_f

if isempty(kx_f)
%     kx_f = abs(F_weight(1))/e_max;
      kx_f = F_max(1)/e_max;
end

if isempty(ky_f)
%     ky_f = abs(F_weight(2))/e_max;
      ky_f = F_max(2)/e_max;
end

if isempty(F_grasp)
    F_grasp = [0;0];
end

if isempty(timeG)
    timeG = 1000;
end

if isempty(kx)
%    kx = max(abs(F_weight(1)), F_max(1))/e_max; 
     kx = F_max(1)/e_max; 
end
if isempty(ky)
%    ky = max(abs(F_weight(2)), F_max(2))/e_max;
     ky = F_max(2)/e_max;
end

% initialization of k and d 
if isempty(kx_i)
%    kx_i = max(abs(F_weight(1)), F_max(1))/e_max; 
     kx_i = kx;
end
if isempty(ky_i)
%    ky_i = max(abs(F_weight(2)), F_max(2))/e_max;
     ky_i = ky;
end
if isempty(dx)
    dx = sqrt(4*kx_i*mass);
end
if isempty(dy)
    dy = sqrt(4*ky_i*mass);
end

% start algoritm with k variable
if comp(1) == 1
    if abs(F_ext(1))/kx > e_max
        if timeG == 1000
            timeG = time;
        end
        kx_f = abs(F_ext(1))/e_max;
        % definition of k_dot for stability condition (from article)
        k_dotx = berta*(4*a0*sqrt(kx_i/mass)*(kx_i)^(3/2))/(sqrt(kx_i) + 2*a0*csi*sqrt(kx_i));
        % law for increasing k
        k_tempx = kx_i + k_dotx*(time -timeG);
        if k_tempx > kx_f
            kx = kx_f;
        else
            kx = k_tempx;
        end
        dx = sqrt(4*kx*mass);
    end
end

if comp(2) == 1
    if abs(F_ext(2))/ky > e_max
        if timeG == 1000
            timeG = time;
        end
        ky_f = abs(F_ext(2))/e_max;
        k_doty = berta*(4*a0*sqrt(ky_i/mass)*(ky_i)^(3/2))/(sqrt(ky_i) + 2*a0*csi*sqrt(ky_i));
        k_tempy = ky_i + k_doty*(time -timeG);
        if k_tempy > ky_f
            ky = ky_f;
        else
            ky = k_tempy;
        end
        dy = sqrt(4*ky*mass);
    end
end

% Final Values of D-K
Kxc = kx;
Kyc = ky;
Dxc = dx;
Dyc = dy;
end

== matlab function tasks_union_1/F_ext2 ==
  data: z input; F_ext output; z_can input; grasping input; mass_can parameter; g parameter
function F_ext = fcn(z, z_can, grasping, mass_can, g)
% hypothesis: table reaction force with elastic behaviour
F_ext = zeros(2,1);
k_can = 500;         
k_table = 10000;
% if contact is happened with can
if grasping == 0
    if z(1) > z_can
        F_ext(1) = k_can*(z_can - z(1));    % force to the left
    end
else 
    F_ext(1) = 0;
    F_ext(2) = -mass_can*g;
    if z(2) < 0
        F_ext(2) = - k_table*z(2);       % in grasping on the table
    else 
        if (abs(k_table*z(2)) < abs(mass_can*g))
            F_ext(2) = -k_table*z(2);
        else 
            F_ext(2) = - mass_can*g;
        end    
    end
end
end

== matlab function tasks_union_1/PLANNER1/INTERPOLATOR OF K AND D  ==
  settings: updateMethod=DISCRETE
  data: time input; K output; kx_f input; ky_f input; D output; e_max parameter; F_max parameter; M parameter; berta parameter; a0 parameter; mass parameter; csi parameter
function [K,D] = fcn(time, kx_f, ky_f, e_max, F_max,M, berta, a0, mass, csi)

persistent kx ky time_prec

if isempty(time_prec)
    time_prec = 0;
end

if isempty(kx)
   kx = F_max(1)/e_max; 
end
if isempty(ky)
   ky = F_max(2)/e_max;
end

% everytime k is increasing in accordance with stability condition
if kx_f <= kx
    kx = kx_f;
else 
    kx_i = kx;
    k_dotx = berta*(4*a0*sqrt(kx_i/mass)*(kx_i)^(3/2))/(sqrt(kx_i) + 2*a0*csi*sqrt(kx_i));
    k_tempx = kx_i + k_dotx*(time -time_prec);
    if k_tempx > kx_f
        kx = kx_f;
    else
        kx = k_tempx;
    end
end

if ky_f <= ky
    ky = ky_f;
else 
    ky_i = ky;
    k_doty = berta*(4*a0*sqrt(ky_i/mass)*(ky_i)^(3/2))/(sqrt(ky_i) + 2*a0*csi*sqrt(ky_i));
    k_tempy = ky_i + k_doty*(time -time_prec);
    if k_tempy > ky_f
        ky = ky_f;
    else
        ky = k_tempy;
    end
end
time_prec = time;

dx = sqrt(4*kx*M);
dy = sqrt(4*ky*M);

D = diag([dx,dy]);
K = diag([kx,ky]);

end

== matlab function tasks_union_1/RR_Model_Joint_Space/GRAVITY ==
  data: q input size=2; G output double size=2; g parameter; l1 parameter; l2 parameter; m1 parameter; m2 parameter
function G = fcn(q,g, l1, l2, m1, m2)


G = [-(l1/2)*cos(q(1))*m1*g - m2*g*(l1*cos(q(1))+(l2/2)*cos(q(1)+q(2))); ...
    -m2*g*(l2/2)*cos(q(1)+q(2))];

end

== matlab function tasks_union_1/RR_Model_Joint_Space/MASS^-1 ==
  data: q input size=2; ddq output size=2; F_tot input double size=2; I1 parameter; I2 parameter; l1 parameter; l2 parameter; m1 parameter; m2 parameter; grasping input; Ic parameter; mass_can parameter
function ddq = fcn(q,F_tot,I1, I2, l1, l2, m1, m2, grasping, Ic, mass_can)

mc = mass_can;

B = [((l1^2)/4)*m1 + I1 + m2*(l1^2) + m2*((l2^2)/4) + m2*l1*l2*cos(q(2)) + I2, m2*(((l1*l2)/2)*cos(q(2)) + (l2^2)/4) + I2; ...
    m2*(((l1*l2)/2)*cos(q(2)) + (l2^2)/4) + I2, m2*(l2^2)/4 + I2];

% if grasping == 1
%     Bc = [mc*((l1^2) + (l2^2) +2*l1*l2*cos(q(2))) + Ic, mc*((l2^2) + l1*l2*cos(q(2))) + Ic; ...
%           mc*((l2^2) + l1*l2*cos(q(2))) + Ic, mc*(l2^2)+ Ic];
%     B = B + Bc;
% end

ddq = B\F_tot;                      % Ftot*M^-1

end

== matlab function tasks_union_1/RR_Model_Joint_Space/MATLAB Function ==
  data: F input size=2; F_ext output double size=2; q input size=2; l1 parameter; l2 parameter
function F_ext = fcn(F,q,l1, l2)


Ja = [-l1*sin(q(1)) - l2*sin(q(1)+q(2)), -l2*sin(q(1)+q(2)); ...
    l1*cos(q(1)) + l2*cos(q(1)+q(2)), l2*cos(q(1)+q(2))];

F_ext = Ja'*F;

end
